simulink model "Assem1"  (R2019a)
settings: Solver=VariableStepAuto  StartTime=0.0  StopTime=10  RelTol=1e-2  AbsTol=1e-2
model workspace: external: MATLAB File C:\Users\dell\Desktop\20232\do_An\New folder (6)\Assem1_DataFile.m (data not in the file)
values from neighbouring files (symbols this model uses):
  s = (2^(1/2)*(ddq0*(tan(q0)^2 + 1) + 2*dq0*tan(q0)*(tan(q0)^2 + 1) - 2^(1/2)*dq1*tan(q1/2)*(tan(q1/2)^2/2 + 1/2)))/(tan(q1/2)^2 + 1)    [tinh_r_dr.m]    (also in trajectory_hinhthang.m = L-0.5*a*(T-t)^2)
undefined symbols (not defined in the file or in its folder): smiData, X, Y, Z
libraries: sm_lib x151, nesl_utility x3, simulink_extras x1
(part 1 of 5)
settings Model: Creator=dell  LastModifiedBy=dell

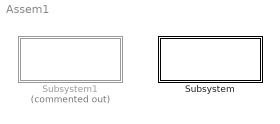
== system Assem1 ==
  Subsystem : Subsystem
  Subsystem1 : Subsystem  Commented=on
